simulink model "emp_filter"  (R2017a)
settings: Solver=VariableStepAuto  StartTime=0.0  StopTime=4  RelTol=1e-3
values from neighbouring files (symbols this model uses):
  step_period = 1    [Init_SNR_sim.m]
  window_size = [50 20 20 20]    [Exp1.mat]    (also in Init_SNR_sim.m = [10 10 10 10])
undefined symbols (not defined in the file or in its folder): magnitude
settings Model: Creator=ignacio  LastModifiedBy=ignacio

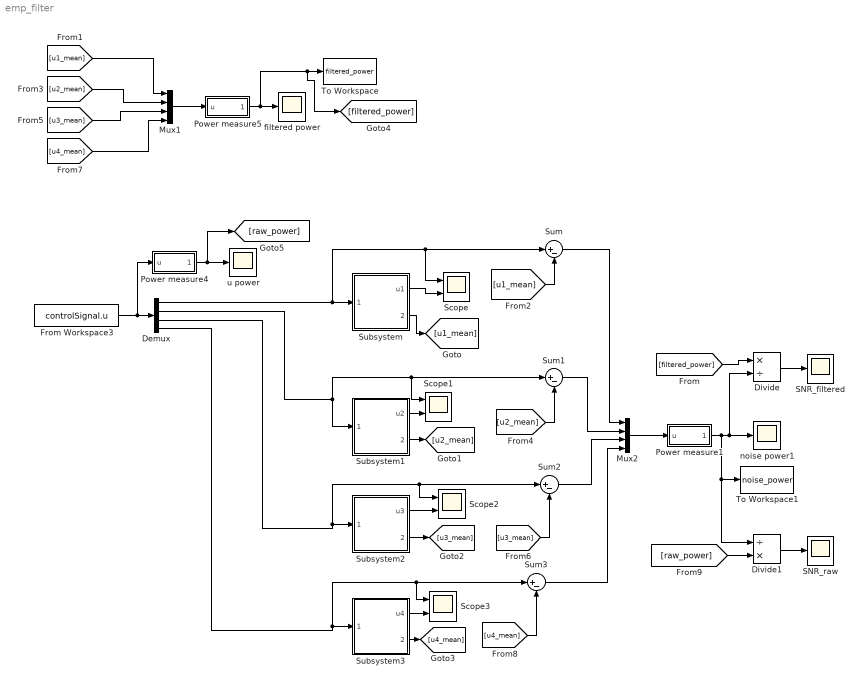
== system emp_filter ==
  Demux : Demux
  Divide : Product  Inputs=*/
  Divide1 : Product  Inputs=/*
  From Workspace3 : FromWorkspace  VariableName=controlSignal.u  SampleTime=0
  Mux1 : Mux
  Mux2 : Mux
  Power measure1 : Subsystem  mask(Measure power){window=0.001, sampling=1e-3}
      mask prompts: window "Window Length"
      mask help: Foo bar
      mask init:
      | global step_period;
      | 
      | N = step_period / window;
  Power measure4 : Subsystem  mask(Measure power){window=0.001, sampling=1e-3}
      mask prompts: window "Window Length"
      mask help: Foo bar
      mask init:
      | global step_period;
      | 
      | N = step_period / window;
  Power measure5 : Subsystem  mask(Measure power){window=0.001, sampling=1e-3}
      mask prompts: window "Window Length"
      mask help: Foo bar
      mask init:
      | global step_period;
      | 
      | N = step_period / window;
  SNR_filtered : Scope
  SNR_raw : Scope
  Scope{,1..3} (4 alike) : Scope  NumInputPorts=2
  Subsystem : Subsystem
  Subsystem1 : Subsystem
  Subsystem2 : Subsystem
  Subsystem3 : Subsystem
  Sum{,1..3} (4 alike) : Sum  Inputs=|+-
  To Workspace : ToWorkspace  VariableName=filtered_power  SaveFormat=Timeseries  SampleTime=-1
  To Workspace1 : ToWorkspace  VariableName=noise_power  SaveFormat=Timeseries  SampleTime=-1
  filtered power : Scope
  noise power1 : Scope
  u power : Scope
  wires:
  Demux/1 -> Sum/1, Scope/1, Subsystem/1(signal)
  Subsystem/1(u1) -> Scope/2
  Subsystem1/1(u2) -> Scope1/2
  Power measure4/1(Power) -> [raw_power], u power/1
  From Workspace3/1 -> Power measure4/1(u), Demux/1
  Mux1/1 -> Power measure5/1(u)
  [u1_mean] -> Mux1/1
  [u2_mean] -> Mux1/2
  [u3_mean] -> Mux1/3
  [u4_mean] -> Mux1/4
  [u1_mean] -> Sum/2
  Demux/2 -> Scope1/1, Sum1/1, Subsystem1/1(signal)
  [u2_mean] -> Sum1/2
  [u3_mean] -> Sum2/2
  Demux/3 -> Subsystem2/1(signal), Scope2/1, Sum2/1
  [u4_mean] -> Sum3/2
  Demux/4 -> Subsystem3/1(signal), Sum3/1, Scope3/1
  Sum/1 -> Mux2/1
  Sum1/1 -> Mux2/2
  Sum2/1 -> Mux2/3
  Sum3/1 -> Mux2/4
  Mux2/1 -> Power measure1/1(u)
  Power measure5/1(Power) -> [filtered_power], To Workspace/1, filtered power/1
  [filtered_power] -> Divide/1
  Divide/1 -> SNR_filtered/1
  Divide1/1 -> SNR_raw/1
  Power measure1/1(Power) -> Divide1/1, To Workspace1/1, Divide/2, noise power1/1
  [raw_power] -> Divide1/2
  Subsystem/2(u1_mean) -> [u1_mean]
  Subsystem1/2(u2_mean) -> [u2_mean]
  Subsystem2/1(u3) -> Scope2/2
  Subsystem2/2(u3_mean) -> [u3_mean]
  Subsystem3/1(u4) -> Scope3/2
  Subsystem3/2(u4_mean) -> [u4_mean]

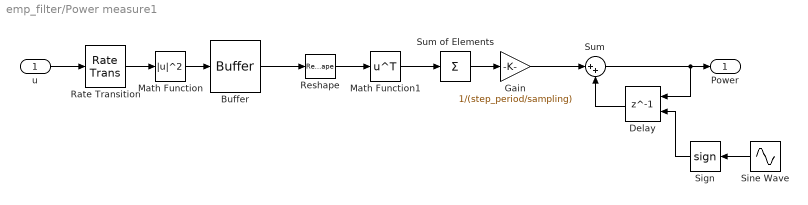
== system emp_filter/Power measure1 ==
  u : Inport
  Buffer : Buffer  N=4* window/sampling  OutputFrames=off
  Delay : Delay  DelayLength=1  ExternalReset=Either
      settings: InputPortMap=u0,r5
  Gain : Gain  Gain=1/(step_period/sampling)
  Math Function : Math  Operator=magnitude^2  SaturateOnIntegerOverflow=on
  Math Function1 : Math  Operator=transpose  SaturateOnIntegerOverflow=on
  Rate Transition : RateTransition  OutPortSampleTime=sampling
  Reshape : Reshape  OutputDimensionality=Customize  OutputDimensions=[4,window/sampling]
  Sign : Signum
  Sine Wave : Sin  Frequency=2*pi / (2 * step_period)  SampleTime=window
  Sum : Sum  Inputs=|++
  Sum of Elements : Sum  Inputs=+  CollapseMode=Specified dimension
  Power : Outport
  wires:
  u/1 -> Rate Transition/1
  Sign/1 -> Delay/2
  Sine Wave/1 -> Sign/1
  Delay/1 -> Sum/2
  Sum/1 -> Power/1, Delay/1
  Math Function1/1 -> Sum of Elements/1
  Buffer/1 -> Reshape/1
  Sum of Elements/1 -> Gain/1
  Reshape/1 -> Math Function1/1
  Gain/1 -> Sum/1
  Rate Transition/1 -> Math Function/1
  Math Function/1 -> Buffer/1

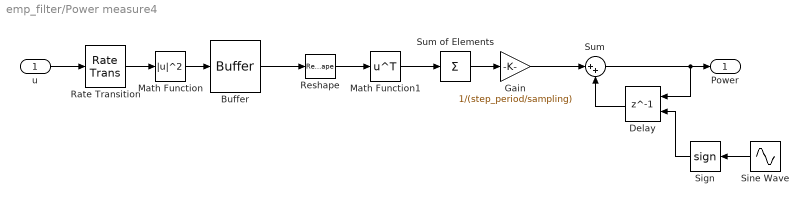
== system emp_filter/Power measure4 ==
  u : Inport
  Buffer : Buffer  N=4* window/sampling  OutputFrames=off
  Delay : Delay  DelayLength=1  ExternalReset=Either
      settings: InputPortMap=u0,r5
  Gain : Gain  Gain=1/(step_period/sampling)
  Math Function : Math  Operator=magnitude^2  SaturateOnIntegerOverflow=on
  Math Function1 : Math  Operator=transpose  SaturateOnIntegerOverflow=on
  Rate Transition : RateTransition  OutPortSampleTime=sampling
  Reshape : Reshape  OutputDimensionality=Customize  OutputDimensions=[4,window/sampling]
  Sign : Signum
  Sine Wave : Sin  Frequency=2*pi / (2 * step_period)  SampleTime=window
  Sum : Sum  Inputs=|++
  Sum of Elements : Sum  Inputs=+  CollapseMode=Specified dimension
  Power : Outport
  wires:
  u/1 -> Rate Transition/1
  Sign/1 -> Delay/2
  Sine Wave/1 -> Sign/1
  Delay/1 -> Sum/2
  Sum/1 -> Power/1, Delay/1
  Math Function1/1 -> Sum of Elements/1
  Buffer/1 -> Reshape/1
  Sum of Elements/1 -> Gain/1
  Reshape/1 -> Math Function1/1
  Gain/1 -> Sum/1
  Rate Transition/1 -> Math Function/1
  Math Function/1 -> Buffer/1

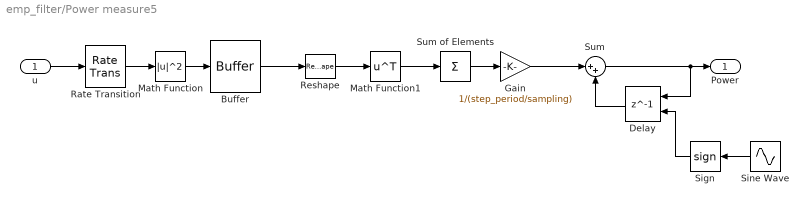
== system emp_filter/Power measure5 ==
  u : Inport
  Buffer : Buffer  N=4* window/sampling  OutputFrames=off
  Delay : Delay  DelayLength=1  ExternalReset=Either
      settings: InputPortMap=u0,r5
  Gain : Gain  Gain=1/(step_period/sampling)
  Math Function : Math  Operator=magnitude^2  SaturateOnIntegerOverflow=on
  Math Function1 : Math  Operator=transpose  SaturateOnIntegerOverflow=on
  Rate Transition : RateTransition  OutPortSampleTime=sampling
  Reshape : Reshape  OutputDimensionality=Customize  OutputDimensions=[4,window/sampling]
  Sign : Signum
  Sine Wave : Sin  Frequency=2*pi / (2 * step_period)  SampleTime=window
  Sum : Sum  Inputs=|++
  Sum of Elements : Sum  Inputs=+  CollapseMode=Specified dimension
  Power : Outport
  wires:
  Math Function/1 -> Buffer/1
  Rate Transition/1 -> Math Function/1
  Gain/1 -> Sum/1
  Reshape/1 -> Math Function1/1
  Sum of Elements/1 -> Gain/1
  Buffer/1 -> Reshape/1
  Math Function1/1 -> Sum of Elements/1
  Sum/1 -> Delay/1, Power/1
  Delay/1 -> Sum/2
  Sine Wave/1 -> Sign/1
  Sign/1 -> Delay/2
  u/1 -> Rate Transition/1

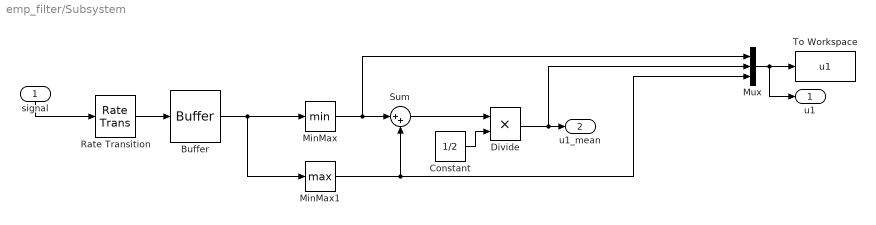
== system emp_filter/Subsystem ==
  signal : Inport
  Buffer : Buffer  N=window_size(1)  V=window_size(1) - 1  OutputFrames=off
  Constant : Constant  Value=1/2
  Divide : Product  SaturateOnIntegerOverflow=on  RndMeth=Zero
  MinMax : MinMax
  MinMax1 : MinMax  Function=max
  Mux : Mux  Inputs=3
  Rate Transition : RateTransition  OutPortSampleTime=simulation_step
  Sum : Sum  Inputs=|++
  To Workspace : ToWorkspace  VariableName=u1  SaveFormat=Timeseries  SampleTime=-1
  u1 : Outport
  u1_mean : Outport  Port=2
  wires:
  MinMax1/1 -> Sum/2, Mux/3
  signal/1 -> Rate Transition/1
  MinMax/1 -> Mux/1, Sum/1
  Sum/1 -> Divide/1
  Divide/1 -> Mux/2, u1_mean/1
  Rate Transition/1 -> Buffer/1
  Constant/1 -> Divide/2
  Buffer/1 -> MinMax1/1, MinMax/1
  Mux/1 -> u1/1, To Workspace/1

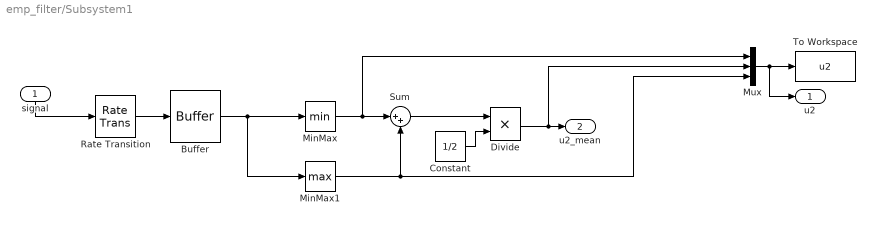
== system emp_filter/Subsystem1 ==
  signal : Inport
  Buffer : Buffer  N=window_size(2)  V=window_size(2) - 1  OutputFrames=off
  Constant : Constant  Value=1/2
  Divide : Product  SaturateOnIntegerOverflow=on  RndMeth=Zero
  MinMax : MinMax
  MinMax1 : MinMax  Function=max
  Mux : Mux  Inputs=3
  Rate Transition : RateTransition  OutPortSampleTime=simulation_step
  Sum : Sum  Inputs=|++
  To Workspace : ToWorkspace  VariableName=u2  SaveFormat=Timeseries  SampleTime=-1
  u2 : Outport
  u2_mean : Outport  Port=2
  wires:
  Mux/1 -> To Workspace/1, u2/1
  Buffer/1 -> MinMax/1, MinMax1/1
  Constant/1 -> Divide/2
  Rate Transition/1 -> Buffer/1
  Divide/1 -> u2_mean/1, Mux/2
  Sum/1 -> Divide/1
  MinMax/1 -> Sum/1, Mux/1
  signal/1 -> Rate Transition/1
  MinMax1/1 -> Mux/3, Sum/2

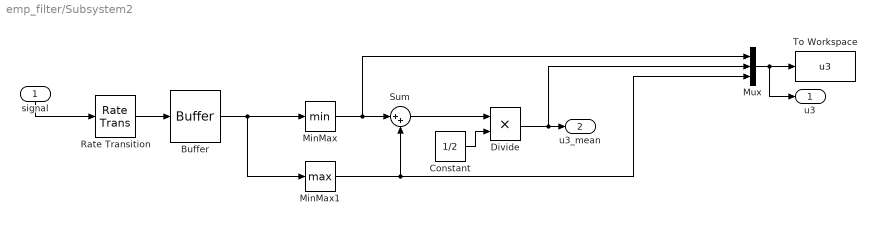
== system emp_filter/Subsystem2 ==
  signal : Inport
  Buffer : Buffer  N=window_size(3)  V=window_size(3) - 1  OutputFrames=off
  Constant : Constant  Value=1/2
  Divide : Product  SaturateOnIntegerOverflow=on  RndMeth=Zero
  MinMax : MinMax
  MinMax1 : MinMax  Function=max
  Mux : Mux  Inputs=3
  Rate Transition : RateTransition  OutPortSampleTime=simulation_step
  Sum : Sum  Inputs=|++
  To Workspace : ToWorkspace  VariableName=u3  SaveFormat=Timeseries  SampleTime=-1
  u3 : Outport
  u3_mean : Outport  Port=2
  wires:
  MinMax1/1 -> Sum/2, Mux/3
  signal/1 -> Rate Transition/1
  MinMax/1 -> Mux/1, Sum/1
  Sum/1 -> Divide/1
  Divide/1 -> Mux/2, u3_mean/1
  Rate Transition/1 -> Buffer/1
  Constant/1 -> Divide/2
  Buffer/1 -> MinMax1/1, MinMax/1
  Mux/1 -> u3/1, To Workspace/1

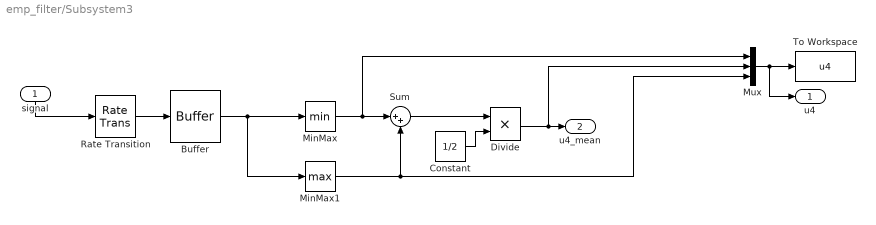
== system emp_filter/Subsystem3 ==
  signal : Inport
  Buffer : Buffer  N=window_size(4)  V=window_size(4) - 1  OutputFrames=off
  Constant : Constant  Value=1/2
  Divide : Product  SaturateOnIntegerOverflow=on  RndMeth=Zero
  MinMax : MinMax
  MinMax1 : MinMax  Function=max
  Mux : Mux  Inputs=3
  Rate Transition : RateTransition  OutPortSampleTime=simulation_step
  Sum : Sum  Inputs=|++
  To Workspace : ToWorkspace  VariableName=u4  SaveFormat=Timeseries  SampleTime=-1
  u4 : Outport
  u4_mean : Outport  Port=2
  wires:
  Mux/1 -> To Workspace/1, u4/1
  Buffer/1 -> MinMax/1, MinMax1/1
  Constant/1 -> Divide/2
  Rate Transition/1 -> Buffer/1
  Divide/1 -> u4_mean/1, Mux/2
  Sum/1 -> Divide/1
  MinMax/1 -> Sum/1, Mux/1
  signal/1 -> Rate Transition/1
  MinMax1/1 -> Mux/3, Sum/2
